simulink model "main"  (R2019b)
settings: Solver=VariableStepAuto  StartTime=0.0  StopTime=0.2  FixedStep=2e-4  RelTol=1e-3
values from neighbouring files (symbols this model uses):
  alpha = 0.2    [RunSim.m]    (also in initSim.m = 0.6; iterationLawFiniteDifference.m = tempAlpha - gamma * J_alpha_square^-1 * J_alpha)
  jerkCoef = 0.0090    (= 0.009)    [RunSim.m]    (also in iterationLawFiniteDifference.m = 0)
  snapCoef = 2.415e-6 + 4.5094e-07    (= 2.86594e-06)    [RunSim.m]    (also in iterationLawFiniteDifference.m = 0)
  Ts = 1/fs    (= 0.0002)    [initSim.m]
libraries: cstblocks x5, simulink x3, dspfdesign x2, model_controller x1
settings Model: Creator=Dai Luyao  LastModifiedBy=Princess
settings DataIOCC: ReturnWorkspaceOutputs=off
settings DebuggingCC: ArithmeticOperatorsInVariantConditions=warning
settings SFSimCC: SimUseLocalCustomCode=off  CustomCodeUndefinedFunction=UseInterfaceOnly
settings RTWCC: RTWUseLocalCustomCode=off
settings CodeAppCC: StateflowObjectComments=on

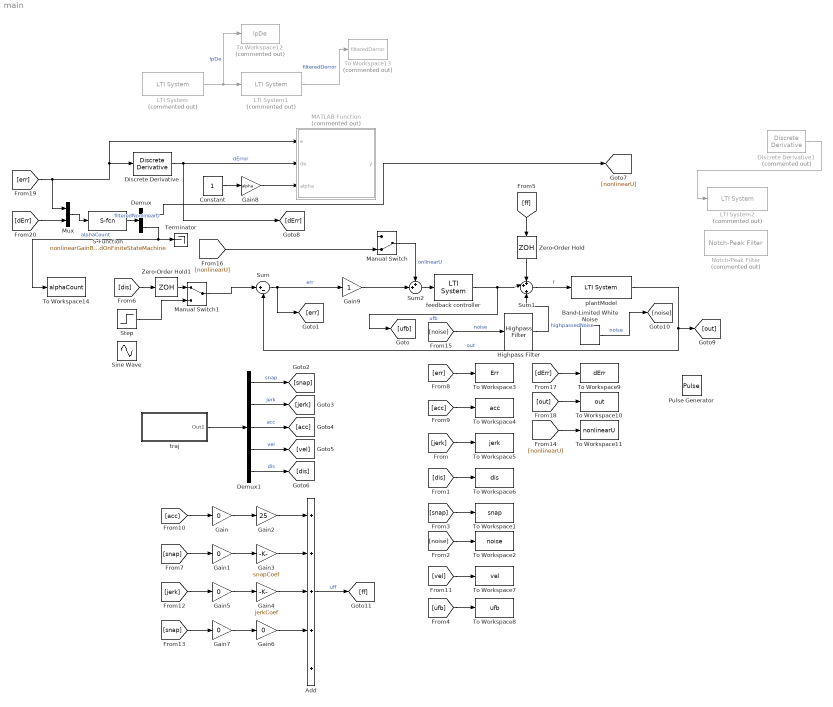
== system main ==
  Add : Sum  Inputs=+++++
  Band-Limited White Noise : simulink/Sources/Band-Limited White Noise  Cov=noisePower  Ts=Ts  seed=[2331]
  Constant : Constant
  Demux : Demux  Outputs=2
  Demux1 : Demux  Outputs=5
  Discrete Derivative : simulink/Discrete/Discrete Derivative  gainval=1.0  ICPrevScaledInput=0.0  OutMin=[]  OutMax=[]  OutDataType=fixdt(1, 16)  OutScaling=2^-10  DoSatur=off
  Discrete Derivative1 : simulink/Discrete/Discrete Derivative  Commented=on  gainval=1.0  ICPrevScaledInput=0.0  OutMin=[]  OutMax=[]  OutDataType=fixdt(1, 16)  OutScaling=2^-10  DoSatur=off
  Gain{,1,5..7} (5 alike) : Gain  Gain=0
  Gain2 : Gain  Gain=25
  Gain3 : Gain  Gain=snapCoef
  Gain4 : Gain  Gain=jerkCoef
  Gain8 : Gain  Gain=alpha
  Gain9 : Gain
  Highpass Filter : dspfdesign/Highpass Filter  FilterType=IIR  DesignForMinimumOrder=off  FilterOrder=4  StopbandFrequency=8e3  PassbandFrequency=400  StopbandAttenuation=80  PassbandRipple=1  InheritSampleRate=off  SampleRate=5000  SimulateUsing=Interpreted execution  roundingMode=Floor  coeffsDataTypeStr=fixdt(1,16)
      settings: SourceProductName=DSP System Toolbox
  LTI System : cstblocks/LTI System  Commented=on  sys=lpFilter  IC=[]
  LTI System1 : cstblocks/LTI System  Commented=on  sys=timeLeadTf  IC=[]
  LTI System2 : cstblocks/LTI System  Commented=on  sys=notchFilter  IC=[]
  MATLAB Function : MATLAB Function  Commented=on  TreatAsAtomicUnit=on
  Manual Switch : ManualSwitch  CurrentSetting=0
  Manual Switch1 : ManualSwitch
  Mux : Mux  Inputs=2
  Notch-Peak Filter : dspfdesign/Notch-Peak Filter  Commented=on  Specification=Bandwidth and center frequency  BandwidthPort=off  Bandwidth=10  QualityFactorPort=off  QualityFactor=5  CenterFrequencyPort=off  CenterFrequency=530  BandwidthCoefficientPort=off  BandwidthCoefficient=0.72654  CenterFrequencyCoefficientPort=off  CenterFrequencyCoefficient=0  Output=Notch and Peak  InheritSampleRate=off  SampleRate=5000  SimulateUsing=Code generation
      settings: SourceProductName=DSP System Toolbox  SourceProductBaseCode=DS
  Pulse Generator : DiscretePulseGenerator  PulseType=Time based  Amplitude=10  Period=0.01  PulseWidth=5
  S-Function : S-Function  FunctionName=nonlinearGainBasedOnFiniteStateMachine  SFunctionDeploymentMode=off  EnableBusSupport=off
  Sine Wave : Sin  Amplitude=30e-6  Frequency=30 * 2 * pi  SampleTime=Ts
  Step : Step  Time=0  After=30e-6  SampleTime=0
  Sum : Sum  Inputs=|+-
  Sum1 : Sum  Inputs=++|+
  Sum2 : Sum  Inputs=++|
  Terminator : Terminator
  To Workspace1 : ToWorkspace  VariableName=snap  SaveFormat=Structure With Time  SampleTime=Ts
  To Workspace10 : ToWorkspace  VariableName=out  SaveFormat=Structure With Time  SampleTime=Ts
  To Workspace11 : ToWorkspace  VariableName=nonlinearU  SaveFormat=Structure With Time  SampleTime=Ts
  To Workspace12 : ToWorkspace  Commented=on  VariableName=lpDe  SaveFormat=Structure With Time  SampleTime=Ts
  To Workspace13 : ToWorkspace  Commented=on  VariableName=filteredDerror  SaveFormat=Structure With Time  SampleTime=Ts
  To Workspace14 : ToWorkspace  VariableName=alphaCount  SaveFormat=Structure With Time  SampleTime=Ts
  To Workspace2 : ToWorkspace  VariableName=noise  SaveFormat=Structure With Time  SampleTime=Ts
  To Workspace3 : ToWorkspace  VariableName=Err  SaveFormat=Structure With Time  SampleTime=Ts
  To Workspace4 : ToWorkspace  VariableName=acc  SaveFormat=Structure With Time  SampleTime=Ts
  To Workspace5 : ToWorkspace  VariableName=jerk  SaveFormat=Structure With Time  SampleTime=Ts
  To Workspace6 : ToWorkspace  VariableName=dis  SaveFormat=Structure With Time  SampleTime=Ts
  To Workspace7 : ToWorkspace  VariableName=vel  SaveFormat=Structure With Time  SampleTime=Ts
  To Workspace8 : ToWorkspace  VariableName=ufb  SaveFormat=Structure With Time  SampleTime=Ts
  To Workspace9 : ToWorkspace  VariableName=dErr  SaveFormat=Structure With Time  SampleTime=Ts
  Zero-Order Hold : ZeroOrderHold  SampleTime=Ts
  Zero-Order Hold1 : ZeroOrderHold  SampleTime=Ts
  feedback controller : cstblocks/LTI System  sys=GcDis  IC=[]
  plantModel : cstblocks/LTI System  sys=GpDis  IC=[]
  traj : Subsystem  BlockChoice=4th order traj
      link override 2nd order traj: x=0.6  v=0.25  a=10
      link override 3rd order traj: j=trajParameters.jerk  v=trajParameters.vel  x=trajParameters.dis  a=trajParameters.acc
      link override 4th order traj: a=trajParameters.acc  v=trajParameters.vel  x=trajParameters.dis  j=trajParameters.jerk  d=trajParameters.snap  Ts=0  t0=0.01
      link override step: vf=1e-6
      settings: AttributesFormatString=%<BlockChoice>  TemplateBlock=model_controller/Profile Generators/traj  MemberBlocks=2th order traj,3rd order traj,4th order traj,step
  wires:
  Sum/1 -> Gain9/1, [err]  "err"
  Demux1/1 -> [snap]  "snap"
  Demux1/2 -> [jerk]  "jerk"
  Demux1/3 -> [acc]  "acc"
  Demux1/4 -> [vel]  "vel"
  Demux1/5 -> [dis]  "dis"
  [acc] -> To Workspace4/1
  [acc] -> Gain/1
  [jerk] -> To Workspace5/1
  [dis] -> To Workspace6/1
  [err] -> To Workspace3/1
  [noise] -> To Workspace2/1
  [ff] -> Zero-Order Hold/1
  [snap] -> To Workspace1/1
  [snap] -> Gain1/1
  Gain/1 -> Gain2/1
  Gain1/1 -> Gain3/1
  Add/1 -> [ff]  "uff"
  Gain2/1 -> Add/1
  Gain3/1 -> Add/2
  [vel] -> To Workspace7/1
  Gain4/1 -> Add/3
  [jerk] -> Gain5/1
  Gain5/1 -> Gain4/1
  Gain7/1 -> Gain6/1
  [snap] -> Gain7/1
  Gain6/1 -> Add/4
  plantModel/1 -> [out], Sum/2  "out"
  traj/1(Out1) -> Demux1/1
  feedback controller/1 -> [ufb], Sum1/2  "ufb"
  Sum1/1 -> plantModel/1  "f"
  [ufb] -> To Workspace8/1
  Zero-Order Hold/1 -> Sum1/1
  Sum2/1 -> feedback controller/1
  Manual Switch/1 -> Sum2/1  "onlinearU"
  Gain8/1 -> MATLAB Function/3(alpha)
  [dis] -> Zero-Order Hold1/1
  Constant/1 -> Gain8/1
  Zero-Order Hold1/1 -> Manual Switch1/1
  Band-Limited White Noise/1 -> [noise]  "noise"
  [dErr] -> To Workspace9/1
  [out] -> To Workspace10/1
  [nonlinearU] -> Manual Switch/2
  Gain9/1 -> Sum2/2
  [nonlinearU] -> To Workspace11/1
  [err] -> Mux/1, Discrete Derivative/1, MATLAB Function/1(e)
  Manual Switch1/1 -> Sum/1
  LTI System/1 -> LTI System1/1, To Workspace12/1  "lpDe"
  Discrete Derivative/1 -> MATLAB Function/2(de), [dErr]  "dError"
  LTI System1/1 -> To Workspace13/1  "filteredDerror"
  [noise] -> Highpass Filter/1  "noise"
  Discrete Derivative1/1 -> LTI System2/1
  [dErr] -> Mux/2
  Mux/1 -> S-Function/1
  S-Function/1 -> Demux/1  "filteredNonlinearU"
  Demux/1 -> [nonlinearU]
  Demux/2 -> Terminator/1, To Workspace14/1  "alphaCount"
  Step/1 -> Manual Switch1/2
  Highpass Filter/1 -> Sum1/3  "highpassedNoise"

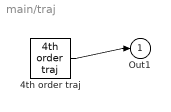
== system main/traj ==
  4th order traj : model_controller/Profile Generators/4th order traj  t0=0.01  x=trajParameters.dis  v=trajParameters.vel  a=trajParameters.acc  j=trajParameters.jerk  d=trajParameters.snap  Ts=0
  Out1 : Outport
  wires:
  4th order traj/1 -> Out1/1

== matlab function main/MATLAB Function ==
  data: e input; y output; de input; alpha input
function y = nonlinearFeedback(e,de,alpha)
%%
% if e*de>0
%     y = alpha * e;
% else
%     y = 0;
% end
%%
global currentErrorState;
global delta;
global currentMin;
global currentMax;

switch currentErrorState
    case ErrorStates.PositiveErrorDown
        if e < currentMin + delta && e > 0
            currentMin = e;
        elseif e < currentMin + delta && e <= 0
            currentMin = e;
            currentErrorState = ErrorStates.NegativeErrorDown;
        else
            currentMax = e;
            currentErrorState = ErrorStates.PositiveErrorUp;
        end
       
        
    case ErrorStates.NegativeErrorDown
        if e < currentMin + delta && e <= 0
            currentMin = e;
        elseif e >= currentMin + delta && e <= 0
            currentMax = e;
            currentErrorState = ErrorStates.NegativeErrorUp;
        else
            currentMax = e;
            currentErrorState = ErrorStates.PositiveErrorUp;
        end
        
        
    case ErrorStates.NegativeErrorUp
        if e > currentMax - delta && e < 0
            currentMax = e;
        elseif e > currentMax - delta && e >= 0
            currentMax = e;
            currentErrorState = ErrorStates.PositiveErrorUp;
        else
            currentMin = e;
            currentErrorState = ErrorStates.NegativeErrorDown;
        end
        
        
    case ErrorStates.PositiveErrorUp
       if e > currentMax - delta && e >= 0
           currentMax = e;
       elseif e <= currentMax - delta && e >=0
           currentMin = e;
           currentErrorState = ErrorStates.PositiveErrorDown;
       else
           currentMin = e;
           currentErrorState = ErrorStates.NegativeErrorDown;
       end
    
    
end

if currentErrorState == ErrorStates.NegativeErrorDown || currentErrorState == ErrorStates.PositiveErrorUp
    y = alpha * e;
else
    y = 0;
end
